simulink model "Trab1_desafio_3"  (R2018a)
settings: Solver=VariableStepAuto  StartTime=0.0  StopTime=10.0  RelTol=1e-6
values from neighbouring files (symbols this model uses):
  inv_Wo = inv_obsv_gramm()    [Trab1_desafio3.m]
  x0 = [0;1;0;-1]    [Trab1_desafio3.m]
undefined symbols (not defined in the file or in its folder): calc_expm
settings Model: Creator=eric-  LastModifiedBy=eric-

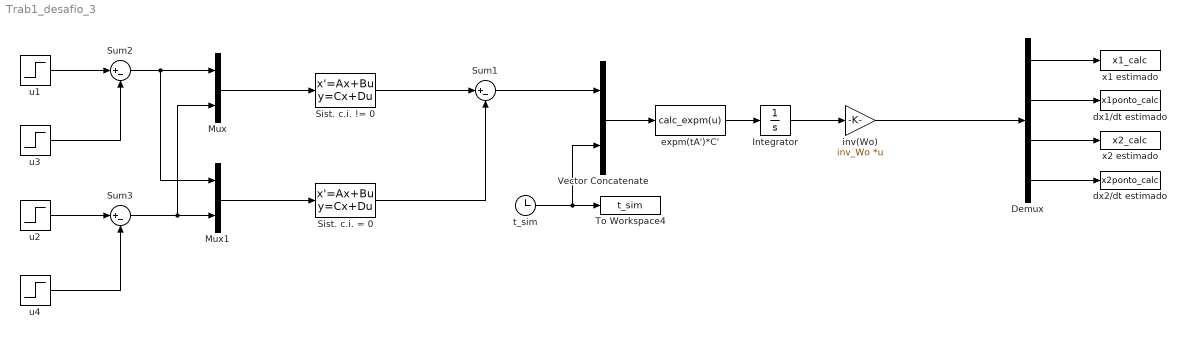
== system Trab1_desafio_3 ==
  Demux : Demux
  Integrator : Integrator
  Mux : Mux  Inputs=2
  Mux1 : Mux  Inputs=2
  Sist. c.i. != 0 : StateSpace  A="[0 1 0 0; -2.25 0 2.25 0;  0 0 0 1; 2.25 0 -2.25 0]"  B=[0 0; 0.25 0; 0 0; 0 0.25]  C=[1 0 0 0; 0 0 1 0]  D=[0 0; 0 0]  InitialCondition=x0
  Sist. c.i. = 0 : StateSpace  A=[0 1 0 0; -2.25 0 2.25 0; 0 0 0 1; 2.25 0 -2.25 0]  B=[0 0; 0.25 0; 0 0; 0 0.25]  C=[1 0 0 0; 0 0 1 0]  D=[0 0; 0 0]  InitialCondition=[0;0;0;0]
  Sum1 : Sum  Inputs=|+-
  Sum2 : Sum  Inputs=|+-
  Sum3 : Sum  Inputs=|+-
  To Workspace4 : ToWorkspace  VariableName=t_sim  SampleTime=-1
      settings: Save2DSignal=2-D array (concatenate along first dimension)
  Vector Concatenate : Concatenate
  dx1/dt estimado : ToWorkspace  VariableName=x1ponto_calc  SampleTime=-1
      settings: Save2DSignal=2-D array (concatenate along first dimension)
  dx2/dt estimado : ToWorkspace  VariableName=x2ponto_calc  SampleTime=-1
      settings: Save2DSignal=2-D array (concatenate along first dimension)
  "expm(tA')*C' " : MATLABFcn  MATLABFcn=calc_expm(u)  Output1D=off
  inv(Wo) : Gain  Gain=inv_Wo  Multiplication=Matrix(K*u)
  t_sim : Clock
  u1 : Step  Time=0  SampleTime=0
  u2 : Step  Time=0  SampleTime=0
  u3 : Step  Time=5  SampleTime=0
  u4 : Step  Time=5  SampleTime=0
  x1 estimado : ToWorkspace  VariableName=x1_calc  SampleTime=-1
      settings: Save2DSignal=2-D array (concatenate along first dimension)
  x2 estimado : ToWorkspace  VariableName=x2_calc  SampleTime=-1
      settings: Save2DSignal=2-D array (concatenate along first dimension)
  wires:
  Sist. c.i. = 0/1 -> Sum1/2
  Sist. c.i. != 0/1 -> Sum1/1
  Mux/1 -> Sist. c.i. != 0/1
  Mux1/1 -> Sist. c.i. = 0/1
  Demux/1 -> x1 estimado/1
  Demux/2 -> dx1/dt estimado/1
  Demux/3 -> x2 estimado/1
  Demux/4 -> dx2/dt estimado/1
  Vector Concatenate/1 -> "expm(tA')*C' "/1
  t_sim/1 -> Vector Concatenate/2, To Workspace4/1
  u1/1 -> Sum2/1
  u3/1 -> Sum2/2
  Sum2/1 -> Mux1/1, Mux/1
  u2/1 -> Sum3/1
  u4/1 -> Sum3/2
  Sum3/1 -> Mux/2, Mux1/2
  Sum1/1 -> Vector Concatenate/1
  "expm(tA')*C' "/1 -> Integrator/1
  Integrator/1 -> inv(Wo)/1
  inv(Wo)/1 -> Demux/1
